simulink model "Processo_PID"  (R2016a)
settings: Solver=VariableStepAuto  StartTime=0.0  StopTime=20  RelTol=1e-3
settings Model: Creator=mende  LastModifiedBy=mende

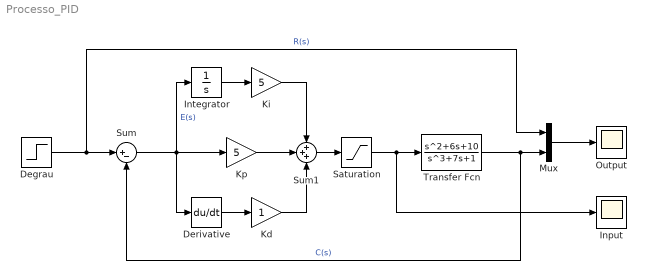
== system Processo_PID ==
  Degrau : Step  SampleTime=0
  Derivative : Derivative
  Input : Scope
  Integrator : Integrator
  Kd : Gain
  Ki : Gain  Gain=5
  Kp : Gain  Gain=5
  Mux : Mux  Inputs=2
  Output : Scope
  Saturation : Saturate  UpperLimit=7  LowerLimit=-7
  Sum : Sum  Inputs=|+-
  Sum1 : Sum  Inputs=+++
  Transfer Fcn : TransferFcn  Numerator=[1,6,10]  Denominator=[1,0,7,1]
  wires:
  Degrau/1 -> Sum/1, Mux/1  "R(s)"
  Transfer Fcn/1 -> Mux/2, Sum/2  "C(s)"
  Sum/1 -> Derivative/1, Integrator/1, Kp/1  "E(s)"
  Mux/1 -> Output/1
  Integrator/1 -> Ki/1
  Sum1/1 -> Saturation/1
  Kp/1 -> Sum1/2
  Ki/1 -> Sum1/1
  Derivative/1 -> Kd/1
  Kd/1 -> Sum1/3
  Saturation/1 -> Input/1, Transfer Fcn/1
